simulink model "pid_model_selector_reset_test"  (R2019b)
settings: Solver=FixedStepAuto  StartTime=0.0  StopTime=20  FixedStep=1e-4  RelTol=1e-3
values from neighbouring files (symbols this model uses):
  B = 0.0002    [pid_values_ziegler_nicholson_manual_vnom_media_agresivo.m]
  J = J_eje + J_carga    (= 0.012)    [pid_values_ziegler_nicholson_manual_vnom_media_agresivo.m]
  Kb = 1.8    [pid_values_ziegler_nicholson_manual_vnom_media_agresivo.m]
  Kd = 0.1    [pid_values_ziegler_nicholson_manual_vnom_media_agresivo.m]
  Ke = 0.025    [pid_values_ziegler_nicholson_manual_vnom_media_agresivo.m]
  Ki = 80    [pid_values_ziegler_nicholson_manual_vnom_media_agresivo.m]
  Kp = 5    [pid_values_ziegler_nicholson_manual_vnom_media_agresivo.m]
  Kt = 1.125    [pid_values_ziegler_nicholson_manual_vnom_media_agresivo.m]
  La = 0.002    [pid_values_ziegler_nicholson_manual_vnom_media_agresivo.m]
  Ra = 0.1    [pid_values_ziegler_nicholson_manual_vnom_media_agresivo.m]
  Td = 0    [pid_values_ziegler_nicholson_manual_vnom_media_agresivo.m]
  V_max = 30    [pid_values_ziegler_nicholson_manual_vnom_media_agresivo.m]
  w_max = 1200    [pid_values_ziegler_nicholson_manual_vnom_media_agresivo.m]
  x_max = 1    [pid_values_ziegler_nicholson_manual_vnom_media_agresivo.m]
  x_min = -1    [pid_values_ziegler_nicholson_manual_vnom_media_agresivo.m]
undefined symbols (not defined in the file or in its folder): sigbuilder_block
libraries: powerlib_meascontrol x1
settings Model: Creator=B00417  LastModifiedBy=B00417
settings SolverCC: ZeroCrossAlgorithm=Adaptive
settings DebuggingCC: IgnoredZcDiagnostic=none

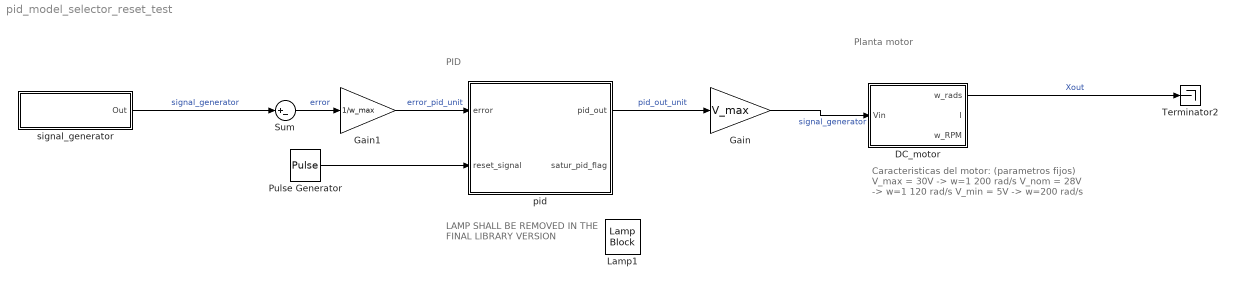
== system pid_model_selector_reset_test ==
  note: Caracteristicas del motor: (parametros fijos)
      | V_max = 30V -> w=1 200 rad/s
      | V_nom = 28V -> w=1 120 rad/s
      | V_min = 5V -> w=200 rad/s
  note: Planta motor
  note: PID
  note: LAMP SHALL BE REMOVED IN THE FINAL LIBRARY VERSION
  DC_motor : Subsystem
      mask Display: disp("M")
  Gain : Gain  Gain=V_max
  Gain1 : Gain  Gain=1/w_max
  Lamp1 : LampBlock
  Pulse Generator : DiscretePulseGenerator  PulseType=Time based  Period=3  PulseWidth=99
  Sum : Sum  Inputs=|+-
  Terminator2 : Terminator
  pid : Subsystem  mask{Kp=Kp, Ki=Ki, Kd=Kd, saturation_off=on, x_max=x_max, x_min=x_min, Ka=Kb}
      mask prompts: Kp "Kp Ganancia proporcional"; Ki "Ki Ganancia integral"; Kd "Kd Ganancia derivativa"; saturation_off "saturation off"; x_max "Salida máxima saturación"; x_min "salida minima satración"; Ka "Ka Ganancia Windup"
      mask init:
      | if Kp < 0
      |     dbstop if Kp<0
      | end
      mask DialogControl wind_up_container Prompt: saturation
      mask Display: disp("PID")
  "signal_generator " : Subsystem  mask{signal=Constant, A=200, f=100, Bias=0, Tstart=0.02, SlewRate=10000, SlewRate_Switch=off}
      mask prompts: A "Amplitude A"; f "Frequency f (Hz)"; Tstart "Start time for step Tstart (s)"; SlewRate "Maximum Slew Rate (1/s)"; SlewRate_Switch "On/Off"
      mask help:
      | Signal_generator
      |
      | Necesita:
      | Entender que es BIOS
      | Saw no funciona (Arreglar)
      |
      | Info:
      | Slew rate es el ratio de subida máximo que permite un generador, generalmente se mide en V/segundo. En este caso, un valor de 1 hace que la pendiente máxima sea 1.
      mask TypeOptions signal: Constant | Step | Sine | Step series | Saw | Builder
      mask Callback signal:
      | 1;
      | 2;
      | 3;
      | 4;
      | 5;
      mask Display: disp('signal_generator')
  wires:
  "signal_generator "/1(Out) -> Sum/1  "signal_generator"
  DC_motor/1(w_rads) -> Terminator2/1  "Xout"
  Sum/1 -> Gain1/1  "error"
  Gain1/1 -> pid/1(error)  "error_pid_unit"
  pid/1(pid_out) -> Gain/1  "pid_out_unit"
  Gain/1 -> DC_motor/1(Vin)  "signal_generator"
  Pulse Generator/1 -> pid/2(reset_signal)

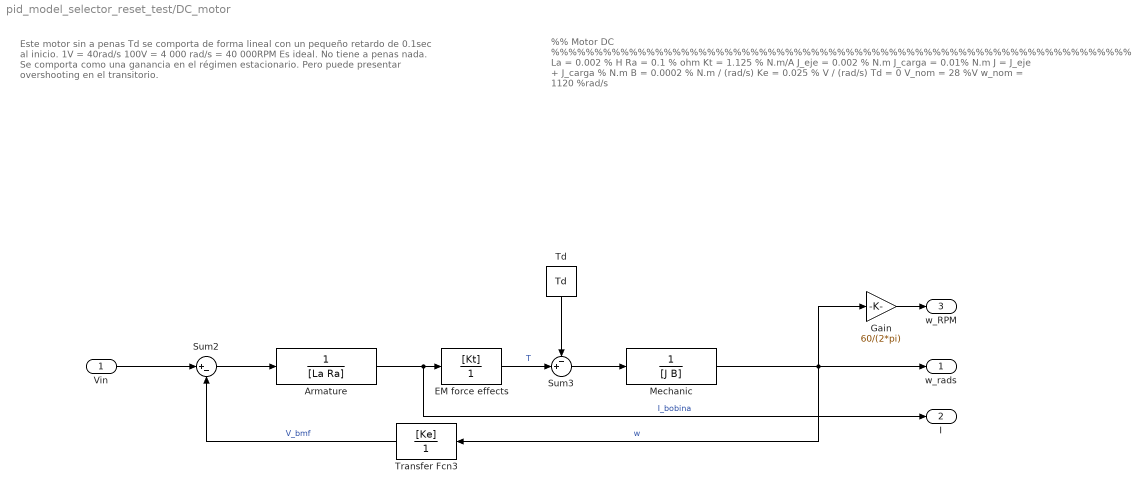
== system pid_model_selector_reset_test/DC_motor ==
  note: Este motor sin a penas Td se comporta de forma lineal con un pequeño retardo de 0.1sec al inicio.
      |
      | 1V = 40rad/s
      | 100V = 4 000 rad/s = 40 000RPM
      | Es ideal. No tiene a penas nada. Se comporta como una ganancia en el régimen estacionario. Pero puede presentar overshooting en el transitorio.
  note: %% Motor DC %%%%%%%%%%%%%%%%%%%%%%%%%%%%%%%%%%%%%%%%%%%%%%%%%%%%%%%%%%%%%%%%%%%
      | La = 0.002 % H
      | Ra = 0.1 % ohm
      | Kt = 1.125 % N.m/A
      | J_eje = 0.002 % N.m
      | J_carga = 0.01% N.m
      | J = J_eje + J_carga % N.m
      | B = 0.0002 % N.m / (rad/s)
      | Ke = 0.025 % V / (rad/s)
      | Td = 0
      | V_nom = 28 %V
      | w_nom = 1120 %rad/s
  Vin : Inport
  Armature : TransferFcn  Denominator=[La Ra]
  "EM force effects " : TransferFcn  Numerator=[Kt]  Denominator=[1]
  Gain : Gain  Gain=60/(2*pi)
  Mechanic : TransferFcn  Denominator=[J B]
  Sum2 : Sum  Inputs=|+-
  Sum3 : Sum  Inputs=-+|
  Td : Constant  Value=Td
  Transfer Fcn3 : TransferFcn  Numerator=[Ke]  Denominator=[1]
  w_rads : Outport
  I : Outport  Port=2
  "w_RPM " : Outport  Port=3
  wires:
  Sum2/1 -> Armature/1
  Sum3/1 -> Mechanic/1
  Armature/1 -> I/1, "EM force effects "/1  "I_bobina"
  Mechanic/1 -> Gain/1, Transfer Fcn3/1, w_rads/1  "w"
  Td/1 -> Sum3/1
  "EM force effects "/1 -> Sum3/2  "T"
  Vin/1 -> Sum2/1
  Transfer Fcn3/1 -> Sum2/2  "V_bmf"
  Gain/1 -> "w_RPM "/1

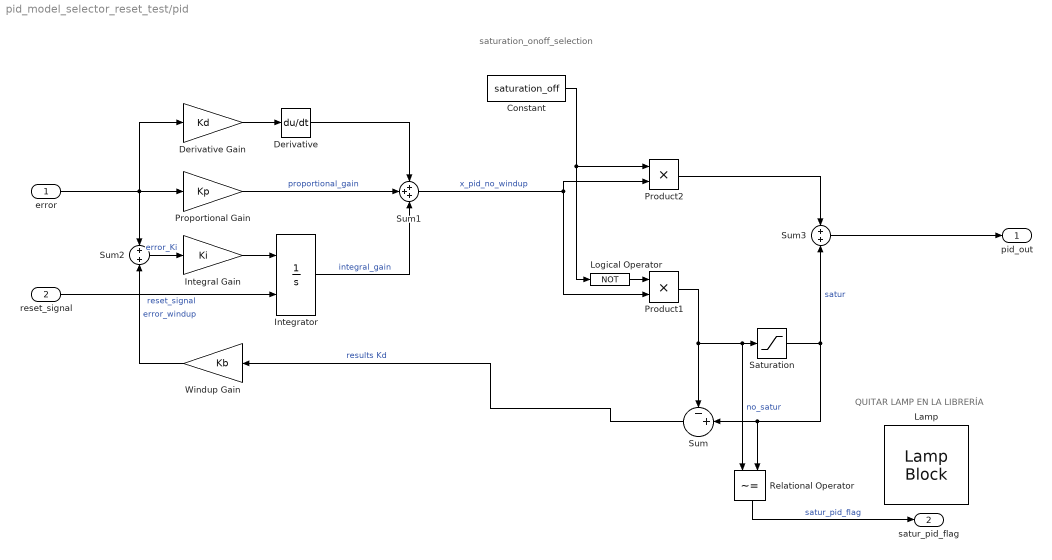
== system pid_model_selector_reset_test/pid ==
  note: QUITAR LAMP EN LA LIBRERÍA
  note: saturation_onoff_selection
  error : Inport
  reset_signal : Inport  Port=2
  Constant : Constant  Value=saturation_off
  Derivative : Derivative
  Derivative Gain : Gain  Gain=Kd
  Integral Gain : Gain  DisableCoverage=on  Gain=Ki
  Integrator : Integrator  ExternalReset=falling
  Lamp : LampBlock
  Logical Operator : Logic  Operator=NOT  AllPortsSameDT=off  OutDataTypeStr=boolean
  Product1 : Product
  Product2 : Product
  Proportional Gain : Gain  Gain=Kp
  Relational Operator : RelationalOperator  Operator=~=  OutDataTypeStr=boolean  RndMeth=Simplest
  Saturation : Saturate  UpperLimit=x_max  LowerLimit=x_min
  Sum : Sum  Inputs=-+|
  Sum1 : Sum  Inputs=+++
  Sum2 : Sum  Inputs=+|+
  Sum3 : Sum  Inputs=+|+
  Windup Gain : Gain  DisableCoverage=on  Gain=Kb
  pid_out : Outport
  satur_pid_flag : Outport  Port=2
  wires:
  Integrator/1 -> Sum1/3  "integral_gain"
  Integral Gain/1 -> Integrator/1
  error/1 -> Derivative Gain/1, Proportional Gain/1, Sum2/1
  Sum1/1 -> Product1/2, Product2/2  "x_pid_no_windup"
  Proportional Gain/1 -> Sum1/2  "proportional_gain"
  reset_signal/1 -> Integrator/2  "reset_signal"
  Saturation/1 -> Sum3/2, Relational Operator/2, Sum/2  "satur"
  Sum2/1 -> Integral Gain/1  "error_Ki"
  Sum/1 -> Windup Gain/1  "results Kd"
  Windup Gain/1 -> Sum2/2  "error_windup"
  Derivative Gain/1 -> Derivative/1
  Derivative/1 -> Sum1/1
  Relational Operator/1 -> satur_pid_flag/1  "satur_pid_flag"
  Sum3/1 -> pid_out/1
  Product2/1 -> Sum3/1
  Product1/1 -> Saturation/1, Relational Operator/1, Sum/1  "no_satur"
  Constant/1 -> Product2/1, Logical Operator/1
  Logical Operator/1 -> Product1/1

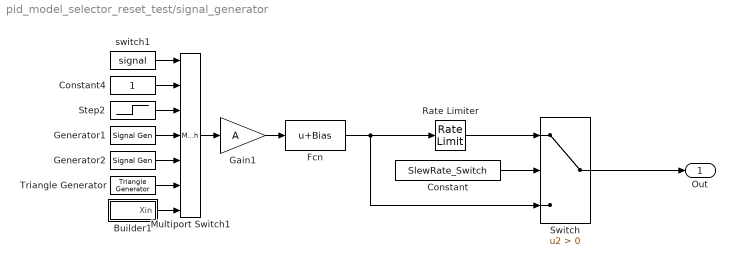
== system pid_model_selector_reset_test/signal_generator  ==
  Builder1 : Subsystem  Tag=STV Subsys  LoadFcn=sigbuilder_block('load');  StartFcn=sigbuilder_block('start');  StopFcn=sigbuilder_block('stop');  ClipboardFcn=sigbuilder_block('clipboard');  mask(Sigbuilder block){tuvar=[0:10]}
      mask help: Simulink:masks:SigbuilderBlock_MD
      mask init:
      | if ~strcmp(get_param(bdroot(gcbh),'SimulationStatus'),'stopped') tuvar = sigbuilder_block('maskInit'); end
      settings: CopyFcn=sigbuilder_block('copy');  DeleteFcn=sigbuilder_block('delete');  ModelCloseFcn=sigbuilder_block('modelClose');  PreSaveFcn=sigbuilder_block('preSave');  PauseFcn=sigbuilder_block('pause')  ContinueFcn=sigbuilder_block('continue')  NameChangeFcn=sigbuilder_block('namechange');  OpenFcn=sigbuilder_block('open',[12 48.75 1213.5 669 ]);  CloseFcn=sigbuilder_block('close');
      mask Display: plot(0, 0, 100, 100,[2, 2, 32, 32, 2], [68, 8, 8, 68, 68],[32, 2], [38, 38], [32, 19, 2],[53, 60, 44], [32, 17, 17, 2],[16, 16, 31, 31]);txt = getActiveGroup(gcbh);text(2, 100, txt,'verticalAlignment', 'top');
  Constant : Constant  Value=SlewRate_Switch
  Constant4 : Constant
  Fcn : Fcn  Expr=u+Bias
  Gain1 : Gain  Gain=A
  Generator1 : SignalGenerator  Frequency=f
      mask Display: disp('Sine')
  Generator2 : SignalGenerator  WaveForm=square  Frequency=f
      mask Display: disp('Square')
  Multiport Switch1 : MultiPortSwitch  Inputs=6
  Rate Limiter : RateLimiter  RisingSlewLimit=SlewRate  FallingSlewLimit=-SlewRate  SampleTimeMode=inherited
  Step2 : Step  Time=Tstart  SampleTime=0
  Switch : Switch  Criteria=u2 > Threshold
  Triangle Generator : powerlib_meascontrol/Pulse & Signal Generators/Triangle Generator  Freq=f  Phase=90  Ts=0
      settings: SourceProductName=Simscape Electrical
  switch1 : Constant  Value=signal
  Out : Outport
  wires:
  Rate Limiter/1 -> Switch/1
  Constant/1 -> Switch/2
  Fcn/1 -> Rate Limiter/1, Switch/3
  Triangle Generator/1 -> Multiport Switch1/6
  Builder1/1(Xin) -> Multiport Switch1/7
  Generator2/1 -> Multiport Switch1/5
  switch1/1 -> Multiport Switch1/1
  Gain1/1 -> Fcn/1
  Multiport Switch1/1 -> Gain1/1
  Step2/1 -> Multiport Switch1/3
  Generator1/1 -> Multiport Switch1/4
  Constant4/1 -> Multiport Switch1/2
  Switch/1 -> Out/1

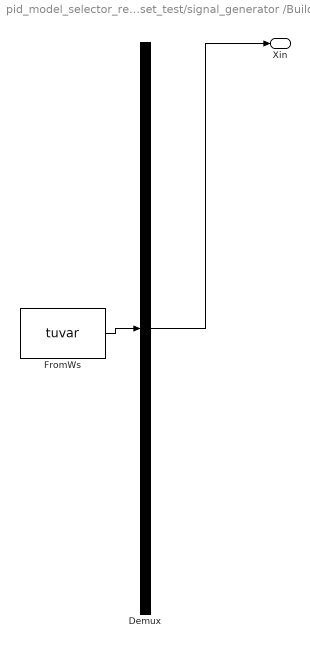
== system pid_model_selector_reset_test/signal_generator /Builder1 ==
  Demux : Demux  Tag=STV Demux  Outputs=1
  FromWs : FromWorkspace  Tag=STV FromWs  VariableName=tuvar  SampleTime=0
      SigBuilderData=|
      | common.afterFinalStr = 'Extrapolate'
      | common.sampleTime = 0
      | dataSet.timeRange = [0 10]
      | dataSet.name = 'Control'
      | sbobj.Groups.Name = 'Control'
      | sbobj.Groups.Signals.Name = 'Xin'
      | sbobj.Groups.Signals.XData = [0 0.1 0.1 1.63 1.63 10]
      | sbobj.Groups.Signals.YData = [0 0 1.01 1.01 -1.015 -0.99]
  Xin : Outport  Tag=STV Outport
  wires:
  Demux/1 -> Xin/1
  FromWs/1 -> Demux/1
